simulink model "SMC_seg_tray_atenuacion_chattering_V1"  (R2026b)
settings: Solver=ode4  StopTime=20  FixedStep=0.0001
settings Model: Creator=nestorhernandezcastellanos  LastModifiedBy=nestorhernandezcastellanos

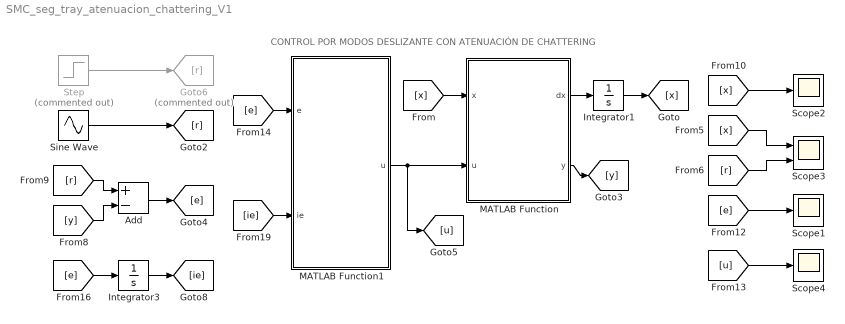
== system SMC_seg_tray_atenuacion_chattering_V1 ==
  note: CONTROL POR MODOS DESLIZANTE CON ATENUACIÓN DE CHATTERING
  Add : Sum  Inputs=+-
  Goto6 : Goto  Commented=on  GotoTag=r
  Integrator1 : Integrator  InitialCondition=1
  Integrator3 : Integrator
  MATLAB Function : MATLAB Function  TreatAsAtomicUnit=on
  MATLAB Function1 : MATLAB Function  TreatAsAtomicUnit=on
  Scope1 : Scope
      settings: ActiveDisplayYMinimum=-1.1345018827917306  ActiveDisplayYMaximum=0.21051694512557476
  Scope2 : Scope
      settings: ActiveDisplayYMinimum=-536580.15017785155  ActiveDisplayYMaximum=343678.24506843346  DataLoggingVariableName=ScopeData2
  Scope3 : Scope  NumInputPorts=2
      settings: ActiveDisplayYMinimum=-1.2503492159106722  ActiveDisplayYMaximum=1.2503463382466187  DataLoggingVariableName=ScopeData3
  Scope4 : Scope
      settings: ActiveDisplayYMinimum=-26.249333606618752  ActiveDisplayYMaximum=26.244002459568783
  Sine Wave : Sin  SampleTime=0
  Step : Step  Commented=on  Time=10  SampleTime=0
  wires:
  MATLAB Function1/1(u) -> [u], MATLAB Function/2(u)
  MATLAB Function/1(dx) -> Integrator1/1
  Sine Wave/1 -> [r]
  [x] -> MATLAB Function/1(x)
  [x] -> Scope3/1
  [r] -> Scope3/2
  Integrator1/1 -> [x]
  MATLAB Function/2(y) -> [y]
  [y] -> Add/2
  [r] -> Add/1
  [e] -> Scope1/1
  [u] -> Scope4/1
  Add/1 -> [e]
  [e] -> MATLAB Function1/1(e)
  Step/1 -> Goto6/1
  [ie] -> MATLAB Function1/2(ie)
  [e] -> Integrator3/1
  Integrator3/1 -> [ie]
  [x] -> Scope2/1

== matlab function SMC_seg_tray_atenuacion_chattering_V1/MATLAB Function1 ==
  data: e input; ie input; u output
function u = controlador(e, ie)

% Ganancia K>1
K = 3;

% Valor arbitrario positivo
m = 4;

Veq = m*abs(e)+2;
sigma = e + m*ie;
u = K*Veq*sign(sigma);

== matlab function SMC_seg_tray_atenuacion_chattering_V1/MATLAB Function ==
  data: x input; dx output; u input; y output
function [dx,y] = planta(x, u)

dx = 2*sin(x)*cos(x) + u;
y = x;
